simulink model "Web_Controlled_PiFace_task"  (Simulink 3.00)
libraries: logiclib x10, mathlib x5, genlib x2, inoutlib x2, execlib x1

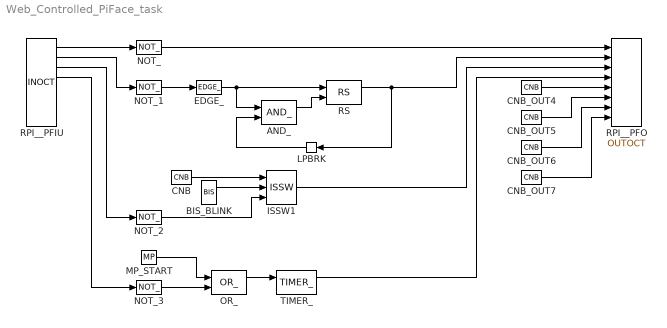
== system Web_Controlled_PiFace_task ==
  AND_ : logiclib/AND_
  BIS_BLINK : genlib/BIS  Y0=off  t1=0.1  t2=0.2  t3=0  t4=4  t5=5  t6=6  t7=7  t8=8  RPT=on
  CNB : mathlib/CNB  YCN=off
  CNB_OUT{4..7} (4 alike) : mathlib/CNB  YCN=off
  EDGE_ : logiclib/EDGE_  iedge=1: Rising edge
  ISSW1 : logiclib/ISSW
  LPBRK : execlib/LPBRK  Orientation=left
  MP_START : genlib/MP  pwidth=1  BSTATE=off  RPTF=off
  NOT_{,1..3} (4 alike) : logiclib/NOT_
  OR_ : logiclib/OR_
  RPI__PFIU : inoutlib/INOCT
  RPI__PFO : inoutlib/OUTOCT
  RS : logiclib/RS
  TIMER_ : logiclib/TIMER_  mode=1: Pulse generator  pt=5
  wires:
  AND_/1 -> RS/2
  BIS_BLINK/1 -> ISSW1/2
  CNB/1 -> ISSW1/1
  CNB_OUT4/1 -> RPI__PFO/5
  CNB_OUT5/1 -> RPI__PFO/6
  CNB_OUT6/1 -> RPI__PFO/7
  CNB_OUT7/1 -> RPI__PFO/8
  EDGE_/1 -> AND_/1, RS/1
  ISSW1/1 -> RPI__PFO/3
  LPBRK/1 -> AND_/2
  MP_START/1 -> OR_/1
  NOT_/1 -> RPI__PFO/1
  NOT_1/1 -> EDGE_/1
  NOT_2/1 -> ISSW1/3
  NOT_3/1 -> OR_/2
  OR_/1 -> TIMER_/1
  RPI__PFIU/1 -> NOT_/1
  RPI__PFIU/2 -> NOT_1/1
  RPI__PFIU/3 -> NOT_2/1
  RPI__PFIU/4 -> NOT_3/1
  RS/1 -> LPBRK/1, RPI__PFO/2
  TIMER_/1 -> RPI__PFO/4
